simulink model "ex4_rs_bsc"  (R2019b)
settings: Solver=FixedStepAuto  StartTime=0  StopTime=100e-3  RelTol=1e-3
model workspace (MAT data in the model file):
  ITV_I = 12
  ITV_M = 17
  M = 4
  RS_k = 188
  RS_m = 8
  RS_n = 204
  RS_prim_poly = 'X^8+X^4+X^3+X^2+1'
  Rb = 1000
  SCR_init = [1 0 0 1 0 1 0 1 0 0 0 0 0 0 0]
  SCR_poly = '1+z^-14+z^-15'
  beta = 0.3
  osf = 16
  span = 12
undefined symbols (not defined in the file or in its folder): rsgenpoly
libraries: commsink2 x2, commblkcod2 x2, commsequence2 x2, commchan3 x1, commrandsrc3 x1
settings Model: Creator=root  LastModifiedBy=E0624826
settings DataIOCC: ReturnWorkspaceOutputs=off
settings DebuggingCC: ArithmeticOperatorsInVariantConditions=warning
settings SFSimCC: SimUseLocalCustomCode=off  CustomCodeUndefinedFunction=UseInterfaceOnly
settings RTWCC: RTWUseLocalCustomCode=off
settings CodeAppCC: StateflowObjectComments=on

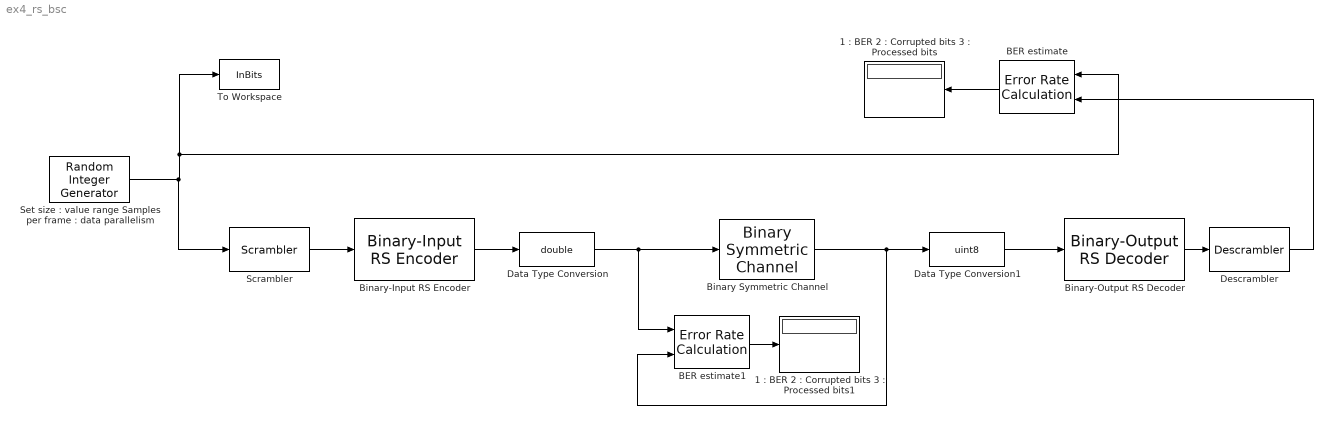
== system ex4_rs_bsc ==
  "1 : BER 2 : Corrupted bits 3 : Processed bits" : Display
  "1 : BER 2 : Corrupted bits 3 : Processed bits1" : Display
  BER estimate : commsink2/Error Rate Calculation  N=0  st_delay=0  cp_mode=Entire frame  subframe=[]  PMode=Port  WsName=ErrorVec  RsMode2=off  stop=off  numErr=100  maxBits=1e6
      settings: SourceProductName=Communications Toolbox
  BER estimate1 : commsink2/Error Rate Calculation  N=0  st_delay=0  cp_mode=Entire frame  subframe=[]  PMode=Port  WsName=ErrorVec  RsMode2=off  stop=off  numErr=100  maxBits=1e6
      settings: SourceProductName=Communications Toolbox
  Binary Symmetric Channel : commchan3/Binary Symmetric Channel  ErrorProbability=1e-3  ErrorVectorOutputPort=off  OutputDataType=double  OutputDataTypeSL=double  Seed=71  SimulateUsing=Code generation
      settings: SourceProductName=Communications Toolbox  SourceProductBaseCode=CM
  Binary-Input RS Encoder : commblkcod2/Binary-Input RS Encoder  n=RS_n  k=RS_k  specShortening=off  shortenedK=3  specGenPoly=on  genPoly=rsgenpoly(2^RS_m-1, 2^RS_m-1-RS_n+RS_k, RS_prim_poly, [], 'double')  specPrimPoly=on  prPoly=RS_prim_poly  specPuncture=off  punctVec=[ones(2,1); zeros(2,1)]  outDType=Same as input
      settings: SourceProductName=Communications Toolbox  SourceProductBaseCode=CM
  Binary-Output RS Decoder : commblkcod2/Binary-Output RS Decoder  n=RS_n  k=RS_k  specShortening=off  shortenedK=3  specGenPoly=on  genPoly=rsgenpoly(2^RS_m-1, 2^RS_m-1-RS_n+RS_k, RS_prim_poly, [], 'double')  specPrimPoly=on  prPoly=RS_prim_poly  specPuncture=off  punctVec=[ones(2,1); zeros(2,1)]  specErasurePort=off  showNumErr=off  outDType=Same as input
      settings: SourceProductName=Communications Toolbox  SourceProductBaseCode=CM
  Data Type Conversion : DataTypeConversion  OutDataTypeStr=double
  Data Type Conversion1 : DataTypeConversion  OutDataTypeStr=uint8
  Descrambler : commsequence2/Descrambler  M=2  poly=SCR_poly  iniStaSource=Dialog Parameter  ini_sta=SCR_init  resetViaPort=off
      settings: SourceProductName=Communications Toolbox  SourceProductBaseCode=CM
  Scrambler : commsequence2/Scrambler  M=2  poly=SCR_poly  iniStaSource=Dialog Parameter  ini_sta=SCR_init  resetViaPort=off
      settings: SourceProductName=Communications Toolbox  SourceProductBaseCode=CM
  "Set size : value range Samples per frame : data parallelism" : commrandsrc3/Random Integer Generator  SetSize=2  SeedSource=Auto  Seed=1922  SampleTime=1/Rb  SamplesPerFrame=RS_k*RS_m*3  OutputDataType=uint8  SimulateUsing=Code generation
      settings: SourceProductName=Communications Toolbox
  To Workspace : ToWorkspace  VariableName=InBits  SaveFormat=Timeseries  SampleTime=-1
  wires:
  "Set size : value range Samples per frame : data parallelism"/1 -> Scrambler/1, To Workspace/1, BER estimate/1
  BER estimate/1 -> "1 : BER 2 : Corrupted bits 3 : Processed bits"/1
  Descrambler/1 -> BER estimate/2
  Scrambler/1 -> Binary-Input RS Encoder/1
  Binary-Output RS Decoder/1 -> Descrambler/1
  BER estimate1/1 -> "1 : BER 2 : Corrupted bits 3 : Processed bits1"/1
  Binary Symmetric Channel/1 -> BER estimate1/2, Data Type Conversion1/1
  Data Type Conversion/1 -> BER estimate1/1, Binary Symmetric Channel/1
  Binary-Input RS Encoder/1 -> Data Type Conversion/1
  Data Type Conversion1/1 -> Binary-Output RS Decoder/1
